simulink model "lars"  (R2021a)
settings: Solver=ode23s  StartTime=0.0  StopTime=10  FixedStep=0.5  RelTol=1e-3
values from neighbouring files (symbols this model uses):
  model =     [untitled.mat]
settings Model: Creator=niezhiwei  LastModifiedBy=niezhiwei
settings SolverCC: ConsecutiveZCsStepRelTol=eps
settings DataIOCC: SaveFinalState=on  SaveFormat=Array  ReturnWorkspaceOutputs=off  SignalLoggingName=sigsout

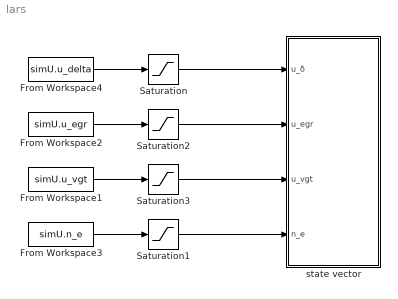
== system lars ==
  From Workspace1 : FromWorkspace  VariableName=simU.u_vgt  Interpolate=off  OutputAfterFinalValue=Holding final value
  From Workspace2 : FromWorkspace  VariableName=simU.u_egr  Interpolate=off  OutputAfterFinalValue=Holding final value
  From Workspace3 : FromWorkspace  VariableName=simU.n_e  Interpolate=off  OutputAfterFinalValue=Holding final value
  From Workspace4 : FromWorkspace  VariableName=simU.u_delta  Interpolate=off  OutputAfterFinalValue=Holding final value
  Saturation : Saturate  UpperLimit=250  LowerLimit=1
  Saturation1 : Saturate  UpperLimit=2000  LowerLimit=500
  Saturation2 : Saturate  UpperLimit=100  LowerLimit=0
  Saturation3 : Saturate  UpperLimit=100  LowerLimit=20
  state vector : Subsystem
  wires:
  Saturation/1 -> state vector/1(u_δ)
  From Workspace4/1 -> Saturation/1
  From Workspace3/1 -> Saturation1/1
  Saturation1/1 -> state vector/4(n_e)
  Saturation2/1 -> state vector/2(u_egr)
  From Workspace2/1 -> Saturation2/1
  Saturation3/1 -> state vector/3(u_vgt)
  From Workspace1/1 -> Saturation3/1

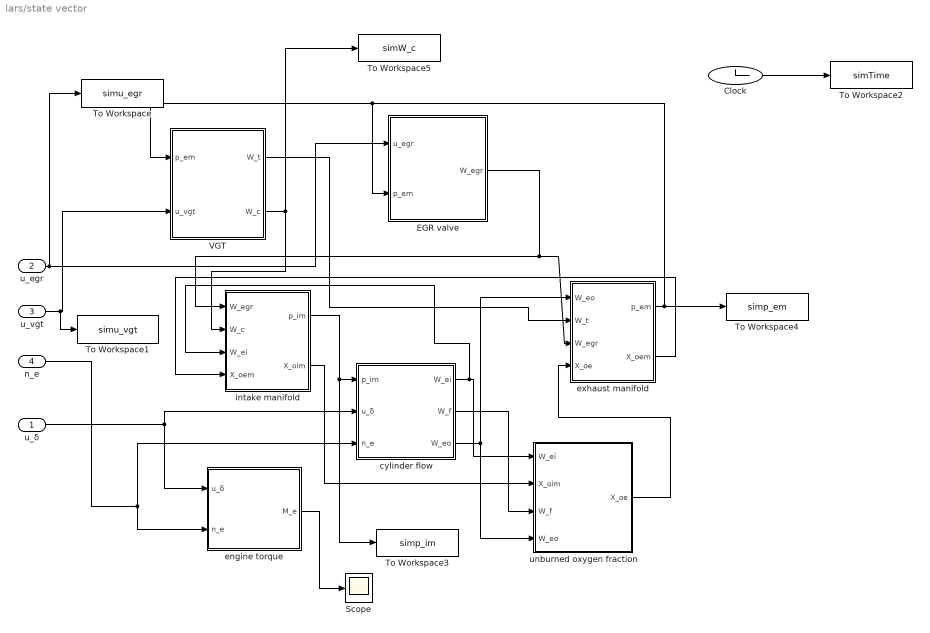
== system lars/state vector ==
  u_δ : Inport
  u_egr : Inport  Port=2
  u_vgt : Inport  Port=3
  n_e : Inport  Port=4
  Clock : Clock
  EGR valve : Subsystem
  Scope : Scope
  To Workspace : ToWorkspace  VariableName=simu_egr  SampleTime=-1
  To Workspace1 : ToWorkspace  VariableName=simu_vgt  SampleTime=-1
  To Workspace2 : ToWorkspace  VariableName=simTime  SampleTime=-1
  To Workspace3 : ToWorkspace  VariableName=simp_im  SampleTime=-1
  To Workspace4 : ToWorkspace  VariableName=simp_em  SampleTime=-1
  To Workspace5 : ToWorkspace  VariableName=simW_c  SampleTime=-1
  VGT : Subsystem
  cylinder flow : Subsystem
  engine torque : Subsystem
  exhaust manifold : Subsystem
  intake manifold : Subsystem
  unburned oxygen fraction : Subsystem
  wires:
  exhaust manifold/2(X_oem) -> intake manifold/4(X_oem)
  u_δ/1 -> engine torque/1(u_δ), cylinder flow/2(u_δ)
  n_e/1 -> engine torque/2(n_e), cylinder flow/3(n_e)
  cylinder flow/2(W_f) -> unburned oxygen fraction/3(W_f)
  intake manifold/2(X_oim) -> unburned oxygen fraction/2(X_oim)
  cylinder flow/1(W_ei) -> unburned oxygen fraction/1(W_ei), intake manifold/3(W_ei)
  cylinder flow/3(W_eo) -> exhaust manifold/1(W_eo), unburned oxygen fraction/4(W_eo)
  EGR valve/1(W_egr) -> intake manifold/1(W_egr), exhaust manifold/3(W_egr)
  VGT/1(W_t) -> exhaust manifold/2(W_t)
  u_vgt/1 -> To Workspace1/1, VGT/2(u_vgt)
  VGT/2(W_c) -> To Workspace5/1, intake manifold/2(W_c)
  unburned oxygen fraction/1(X_oe) -> exhaust manifold/4(X_oe)
  u_egr/1 -> To Workspace/1, EGR valve/1(u_egr)
  Clock/1 -> To Workspace2/1
  intake manifold/1(p_im) -> To Workspace3/1, cylinder flow/1(p_im)
  exhaust manifold/1(p_em) -> EGR valve/2(p_em), VGT/1(p_em), To Workspace4/1
  engine torque/1(M_e) -> Scope/1

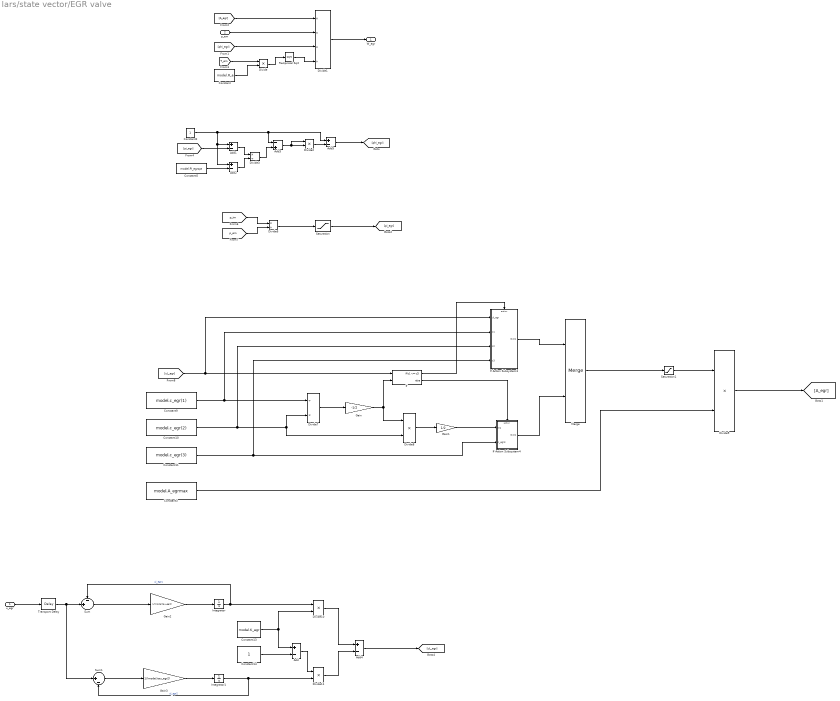
== system lars/state vector/EGR valve ==
  u_egr : Inport
  p_em : Inport  Port=2
  Add{,1..2,4..5} (5 alike) : Sum  Inputs=+-
  Add3 : Sum  Inputs=-+
  Constant : Constant  Value=model.R_e
  Constant10 : Constant  Value=model.c_egr(2)
  Constant11 : Constant  Value=model.c_egr(3)
  Constant13 : Constant  Value=model.K_egr
  Constant14 : Constant
  Constant2 : Constant
  Constant3 : Constant  Value=model.A_egrmax
  Constant5 : Constant  Value=model.PI_egropt
  Constant9 : Constant  Value=model.c_egr(1)
  Divide{,2,8..11} (6 alike) : Product  Inputs=**
  Divide1 : Product  Inputs=***/
  Divide3 : Product  Inputs=*/
  Divide6 : Product  Inputs=*/
  Divide7 : Product  Inputs=/*
  Gain : Gain  Gain=-1/2
  Gain1 : Gain  Gain=1/2
  Gain2 : Gain  Gain=1/(model.tau_egr1)
  Gain3 : Gain  Gain=1/(model.tau_egr2)
  If : If  NumInputs=2  IfExpression=u1 <= u2
  If Action Subsystem3 : Subsystem  TreatAsAtomicUnit=on
  If Action Subsystem4 : Subsystem  TreatAsAtomicUnit=on
  Integrator : Integrator  InitialCondition=model.uInit_egr
  Integrator1 : Integrator  InitialCondition=model.uInit_egr
  Merge : Merge
  Reciprocal Sqrt : Sqrt  SaturateOnIntegerOverflow=on
  Saturation : Saturate  UpperLimit=1  LowerLimit=model.PI_egropt
  Saturation1 : Saturate  UpperLimit=inf  LowerLimit=0
  Sum : Sum  Inputs=-+|
  Sum1 : Sum  Inputs=|+-
  Transport Delay : TransportDelay  DelayTime=model.tau_degr  InitialOutput=model.uInit_egr
  W_egr : Outport
  wires:
  [T_em] -> Divide/1
  Constant/1 -> Divide/2
  Divide/1 -> Reciprocal Sqrt/1
  [phi_egr] -> Divide1/3
  p_em/1 -> Divide1/2
  [A_egr] -> Divide1/1
  Reciprocal Sqrt/1 -> Divide1/4
  [pi_egr] -> Add1/2
  Constant2/1 -> Add2/1, Add1/1, Add5/1, Add3/1
  Constant5/1 -> Add2/2
  Add2/1 -> Divide3/2
  Add1/1 -> Divide3/1
  Divide3/1 -> Add3/2
  Add3/1 -> Divide2/1, Divide2/2
  Divide2/1 -> Add5/2
  Add5/1 -> [phi_egr]
  [p_im] -> Divide6/1
  [p_em] -> Divide6/2
  Divide1/1 -> W_egr/1
  Constant10/1 -> If Action Subsystem3/3(c2), Divide7/2, Divide8/2
  Constant9/1 -> If Action Subsystem3/2(c1), Divide7/1
  Divide7/1 -> Gain/1
  Gain/1 -> If/2, Divide8/1
  [uL_egr] -> If Action Subsystem3/1(ul_egr), If/1
  Constant11/1 -> If Action Subsystem3/4(c3), If Action Subsystem4/2(c_egr3)
  Divide8/1 -> Gain1/1
  Gain1/1 -> If Action Subsystem4/1(In1)
  Constant3/1 -> Divide9/2
  Divide9/1 -> [A_egr]
  Integrator/1 -> Divide10/1, Sum/1  "ul_egr1"
  Constant13/1 -> Add/1, Divide10/2
  Constant14/1 -> Add/2
  Integrator1/1 -> Sum1/2, Divide11/2  "ul_egr2"
  Add/1 -> Divide11/1
  Divide10/1 -> Add4/1
  Divide11/1 -> Add4/2
  Add4/1 -> [uL_egr]
  Gain2/1 -> Integrator/1
  Sum/1 -> Gain2/1
  Sum1/1 -> Gain3/1
  Gain3/1 -> Integrator1/1
  u_egr/1 -> Transport Delay/1
  Transport Delay/1 -> Sum/2, Sum1/1
  Saturation/1 -> [pi_egr]
  Divide6/1 -> Saturation/1
  If/2 -> If Action Subsystem4/Action
  If/1 -> If Action Subsystem3/Action
  Merge/1 -> Saturation1/1
  If Action Subsystem3/1(Out1) -> Merge/1
  If Action Subsystem4/1(Out1) -> Merge/2
  Saturation1/1 -> Divide9/1

== system lars/state vector/VGT ==
  p_em : Inport
  u_vgt : Inport  Port=2
  To Workspace3 : ToWorkspace  VariableName=W_c  SampleTime=-1
  compressor : Subsystem
  turbo : Subsystem
  W_t : Outport
  W_c : Outport  Port=2
  wires:
  turbo/1(W_t) -> W_t/1
  u_vgt/1 -> turbo/1(u_vgt)
  compressor/1(W_c) -> W_c/1, To Workspace3/1
  turbo/2(omega_t) -> compressor/1(omega_t)
  p_em/1 -> turbo/2(p_em)
  compressor/2(P_c) -> turbo/3(P_c)

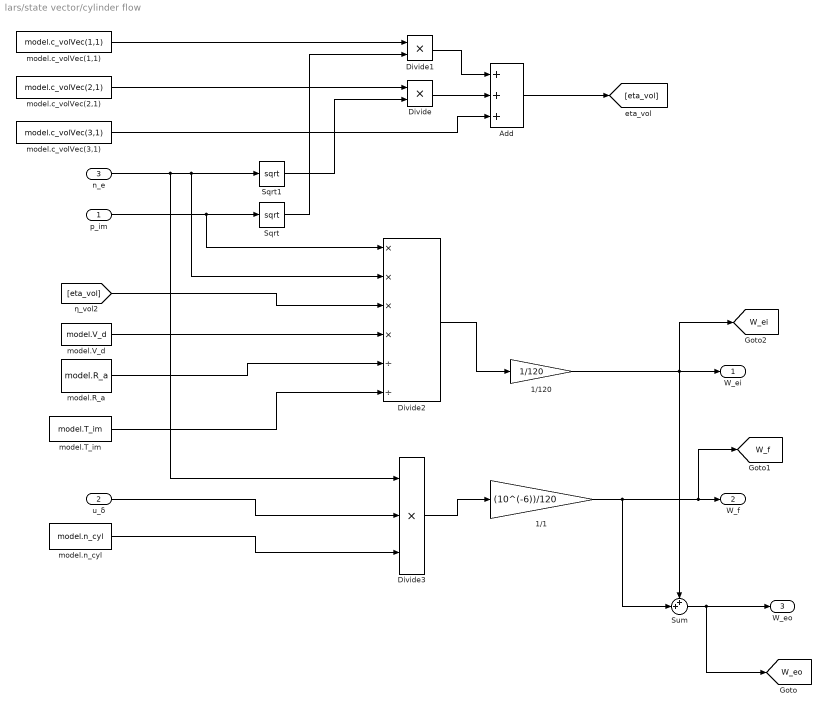
== system lars/state vector/cylinder flow ==
  p_im : Inport
  u_δ : Inport  Port=2
  n_e : Inport  Port=3
  1/1 : Gain  Gain=(10^(-6))/120
  1/120 : Gain  Gain=1/120
  Add : Sum  Inputs=+++
  Divide : Product  Inputs=**
  Divide1 : Product  Inputs=**
  Divide2 : Product  Inputs=****//
  Divide3 : Product  Inputs=***
  Sqrt : Sqrt  SaturateOnIntegerOverflow=on
  Sqrt1 : Sqrt  SaturateOnIntegerOverflow=on
  Sum : Sum  Inputs=++|
  model.R_a : Constant  Value=model.R_a
  model.T_im : Constant  Value=model.T_im
  model.V_d : Constant  Value=model.V_d
  model.c_volVec(1,1) : Constant  Value=model.c_volVec(1,1)
  model.c_volVec(2,1) : Constant  Value=model.c_volVec(2,1)
  model.c_volVec(3,1) : Constant  Value=model.c_volVec(3,1)
  model.n_cyl : Constant  Value=model.n_cyl
  W_ei : Outport
  W_f : Outport  Port=2
  W_eo : Outport  Port=3
  tag scope: W_ei=global, W_eo=global, W_f=global
  wires:
  p_im/1 -> Divide2/1, Sqrt/1
  n_e/1 -> Divide3/1, Divide2/2, Sqrt1/1
  model.c_volVec(2,1)/1 -> Divide/1
  model.c_volVec(1,1)/1 -> Divide1/1
  Sqrt/1 -> Divide1/2
  Divide1/1 -> Add/1
  Divide/1 -> Add/2
  model.c_volVec(3,1)/1 -> Add/3
  Add/1 -> [eta_vol]
  [eta_vol] -> Divide2/3
  model.V_d/1 -> Divide2/4
  model.R_a/1 -> Divide2/5
  model.T_im/1 -> Divide2/6
  Divide2/1 -> 1/120/1
  1/120/1 -> [W_ei], Sum/1, W_ei/1
  u_δ/1 -> Divide3/2
  model.n_cyl/1 -> Divide3/3
  Divide3/1 -> 1/1/1
  1/1/1 -> Sum/2, [W_f], W_f/1
  Sum/1 -> [W_eo], W_eo/1
  Sqrt1/1 -> Divide/2

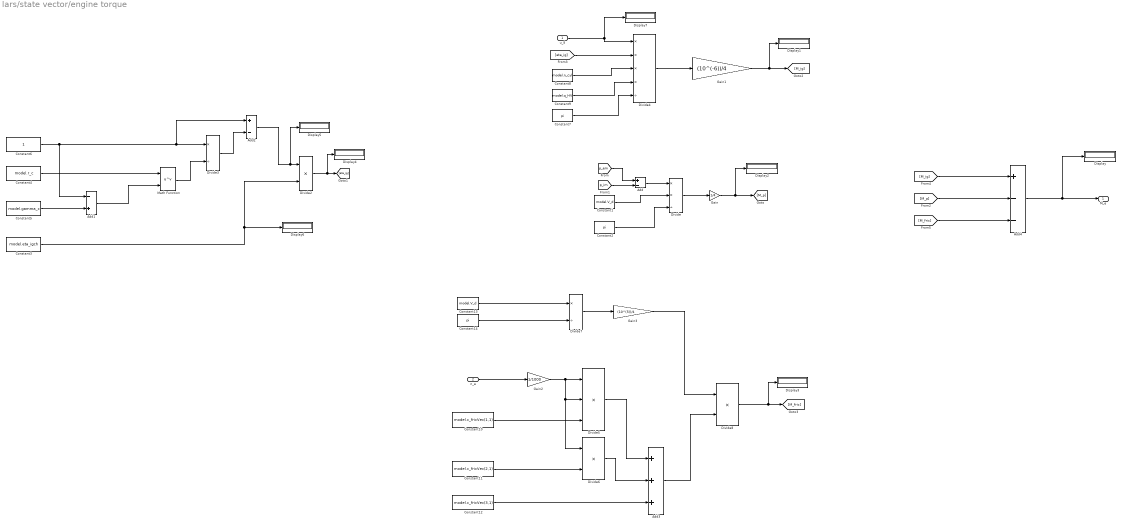
== system lars/state vector/engine torque ==
  u_δ : Inport
  n_e : Inport  Port=2
  Add : Sum  Inputs=+-
  Add1 : Sum  Inputs=-+
  Add2 : Sum  Inputs=+-
  Add3 : Sum  Inputs=+++
  Add4 : Sum  Inputs=+--
  Constant1 : Constant  Value=model.V_d
  Constant10 : Constant  Value=model.c_fricVec(1,1)
  Constant11 : Constant  Value=model.c_fricVec(2,1)
  Constant12 : Constant  Value=model.c_fricVec(3,1)
  Constant13 : Constant  Value=model.V_d
  Constant14 : Constant  Value=pi
  Constant2 : Constant  Value=pi
  Constant3 : Constant  Value=model.eta_igch
  Constant4 : Constant  Value=model.r_c
  Constant5 : Constant  Value=model.gamma_c
  Constant6 : Constant
  Constant7 : Constant  Value=pi
  Constant8 : Constant  Value=model.n_cyl
  Constant9 : Constant  Value=model.q_HV
  Display{,1..7} (8 alike) : Display
  Divide : Product  Inputs=**/
  Divide2 : Product  Inputs=**
  Divide3 : Product  Inputs=*/
  Divide4 : Product  Inputs=****/
  Divide5 : Product  Inputs=***
  Divide6 : Product  Inputs=**
  Divide7 : Product  Inputs=*/
  Divide8 : Product  Inputs=**
  Gain : Gain  Gain=1/4
  Gain1 : Gain  Gain=(10^(-6))/4
  Gain2 : Gain  Gain=1/1000
  Gain3 : Gain  Gain=(10^(5))/4
  Math Function : Math  Operator=pow  SaturateOnIntegerOverflow=on
  M_e : Outport
  wires:
  [p_em] -> Add/1
  [p_im] -> Add/2
  Add/1 -> Divide/1
  Constant1/1 -> Divide/2
  Constant2/1 -> Divide/3
  Divide/1 -> Gain/1
  Constant6/1 -> Add1/1, Add2/1, Divide3/1
  Constant4/1 -> Math Function/1
  Math Function/1 -> Divide3/2
  Divide3/1 -> Add2/2
  Constant3/1 -> Display6/1, Divide2/2
  Add2/1 -> Display5/1, Divide2/1
  Divide2/1 -> Display4/1, [eta_ig]
  u_δ/1 -> Display7/1, Divide4/1
  [eta_ig] -> Divide4/2
  Constant8/1 -> Divide4/3
  Constant9/1 -> Divide4/4
  Constant7/1 -> Divide4/5
  Divide4/1 -> Gain1/1
  Gain1/1 -> Display1/1, [M_ig]
  n_e/1 -> Gain2/1
  Gain2/1 -> Divide5/1, Divide5/2, Divide6/1
  Constant10/1 -> Divide5/3
  Constant11/1 -> Divide6/2
  Divide5/1 -> Add3/1
  Divide6/1 -> Add3/2
  Constant12/1 -> Add3/3
  Constant13/1 -> Divide7/1
  Constant14/1 -> Divide7/2
  Divide7/1 -> Gain3/1
  Gain3/1 -> Divide8/1
  Add3/1 -> Divide8/2
  Divide8/1 -> Display3/1, [M_fric]
  [M_ig] -> Add4/1
  [M_p] -> Add4/2
  [M_fric] -> Add4/3
  Add4/1 -> Display/1, M_e/1
  Gain/1 -> Display2/1, [M_p]
  Constant5/1 -> Add1/2
  Add1/1 -> Math Function/2

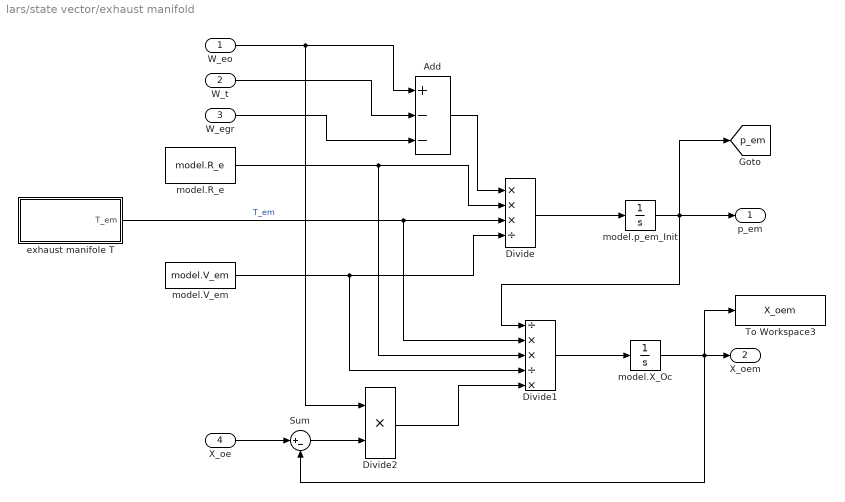
== system lars/state vector/exhaust manifold ==
  W_eo : Inport
  W_t : Inport  Port=2
  W_egr : Inport  Port=3
  X_oe : Inport  Port=4
  Add : Sum  Inputs=+--
  Divide : Product  Inputs=***/
  Divide1 : Product  Inputs=/**/*
  Divide2 : Product  Inputs=**
  Sum : Sum  Inputs=|+-
  To Workspace3 : ToWorkspace  VariableName=X_oem  SampleTime=-1
  exhaust manifole T : Subsystem
  model.R_e : Constant  Value=model.R_e
  model.V_em : Constant  Value=model.V_em
  model.X_Oc : Integrator  LimitOutput=on  UpperSaturationLimit=1  LowerSaturationLimit=0
  model.p_em_Init : Integrator  InitialCondition=model.p_em_Init  LimitOutput=on  UpperSaturationLimit=20*model.p_amb  LowerSaturationLimit=0.5*model.p_amb
  p_em : Outport
  X_oem : Outport  Port=2
  tag scope: p_em=global
  wires:
  model.p_em_Init/1 -> Divide1/1, [p_em], p_em/1
  model.R_e/1 -> Divide1/3, Divide/2
  exhaust manifole T/1(T_em) -> Divide/3, Divide1/2  "T_em"
  model.V_em/1 -> Divide1/4, Divide/4
  Add/1 -> Divide/1
  W_egr/1 -> Add/3
  W_t/1 -> Add/2
  W_eo/1 -> Add/1, Divide2/1
  Divide1/1 -> model.X_Oc/1
  X_oe/1 -> Sum/1
  Divide2/1 -> Divide1/5
  Sum/1 -> Divide2/2
  Divide/1 -> model.p_em_Init/1
  model.X_Oc/1 -> To Workspace3/1, Sum/2, X_oem/1

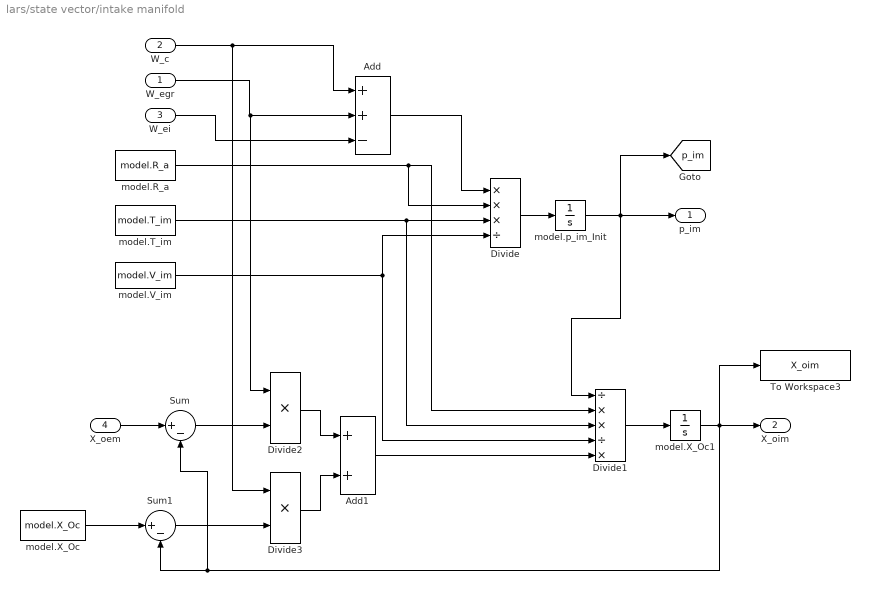
== system lars/state vector/intake manifold ==
  W_egr : Inport
  W_c : Inport  Port=2
  W_ei : Inport  Port=3
  X_oem : Inport  Port=4
  Add : Sum  Inputs=++-
  Add1 : Sum
  Divide : Product  Inputs=***/
  Divide1 : Product  Inputs=/**/*
  Divide2 : Product  Inputs=**
  Divide3 : Product  Inputs=**
  Sum : Sum  Inputs=|+-
  Sum1 : Sum  Inputs=|+-
  To Workspace3 : ToWorkspace  VariableName=X_oim  SampleTime=-1
  model.R_a : Constant  Value=model.R_a
  model.T_im : Constant  Value=model.T_im
  model.V_im : Constant  Value=model.V_im
  model.X_Oc : Constant  Value=model.X_Oc
  model.X_Oc1 : Integrator  LimitOutput=on  UpperSaturationLimit=1  LowerSaturationLimit=0
  model.p_im_Init : Integrator  InitialCondition=model.p_im_Init  LimitOutput=on  UpperSaturationLimit=10*model.p_amb  LowerSaturationLimit=0.5*model.p_amb
  p_im : Outport
  X_oim : Outport  Port=2
  tag scope: p_im=global
  wires:
  W_egr/1 -> Divide2/1, Add/2
  W_ei/1 -> Add/3
  Add/1 -> Divide/1
  model.V_im/1 -> Divide/4, Divide1/4
  model.T_im/1 -> Divide/3, Divide1/3
  model.R_a/1 -> Divide1/2, Divide/2
  Divide/1 -> model.p_im_Init/1
  model.p_im_Init/1 -> Divide1/1, [p_im], p_im/1
  Divide1/1 -> model.X_Oc1/1
  X_oem/1 -> Sum/1
  model.X_Oc/1 -> Sum1/1
  Sum/1 -> Divide2/2
  Sum1/1 -> Divide3/2
  Divide2/1 -> Add1/1
  Divide3/1 -> Add1/2
  Add1/1 -> Divide1/5
  W_c/1 -> Add/1, Divide3/1
  model.X_Oc1/1 -> To Workspace3/1, Sum1/2, Sum/2, X_oim/1

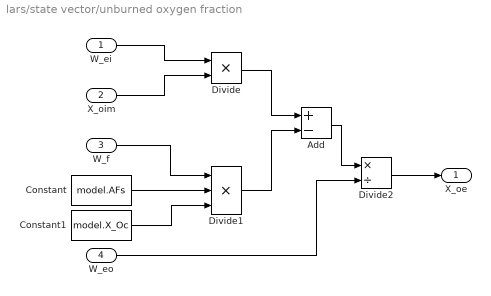
== system lars/state vector/unburned oxygen fraction ==
  W_ei : Inport
  X_oim : Inport  Port=2
  W_f : Inport  Port=3
  W_eo : Inport  Port=4
  Add : Sum  Inputs=+-
  Constant : Constant  Value=model.AFs
  Constant1 : Constant  Value=model.X_Oc
  Divide : Product  Inputs=**
  Divide1 : Product  Inputs=***
  Divide2 : Product  Inputs=*/
  X_oe : Outport
  wires:
  X_oim/1 -> Divide/2
  W_f/1 -> Divide1/1
  Constant/1 -> Divide1/2
  Divide/1 -> Add/1
  Divide1/1 -> Add/2
  Add/1 -> Divide2/1
  W_eo/1 -> Divide2/2
  Divide2/1 -> X_oe/1
  W_ei/1 -> Divide/1
  Constant1/1 -> Divide1/3

== system lars/state vector/EGR valve/If Action Subsystem3 ==
  ul_egr : Inport
  c1 : Inport  Port=2
  c2 : Inport  Port=3
  c3 : Inport  Port=4
  Action Port : ActionPort  ActionPortLabel=if(u1 <= u2)
  Add : Sum  Inputs=+++
  Divide : Product  Inputs=***
  Divide1 : Product  Inputs=**
  Out1 : Outport
  wires:
  ul_egr/1 -> Divide1/1, Divide/2, Divide/1
  c1/1 -> Divide/3
  c2/1 -> Divide1/2
  Divide/1 -> Add/1
  Divide1/1 -> Add/2
  c3/1 -> Add/3
  Add/1 -> Out1/1

== system lars/state vector/EGR valve/If Action Subsystem4 ==
  In1 : Inport
  c_egr3 : Inport  Port=2
  Action Port : ActionPort  ActionPortLabel=else
  Add : Sum
  Out1 : Outport
  wires:
  In1/1 -> Add/1
  c_egr3/1 -> Add/2
  Add/1 -> Out1/1

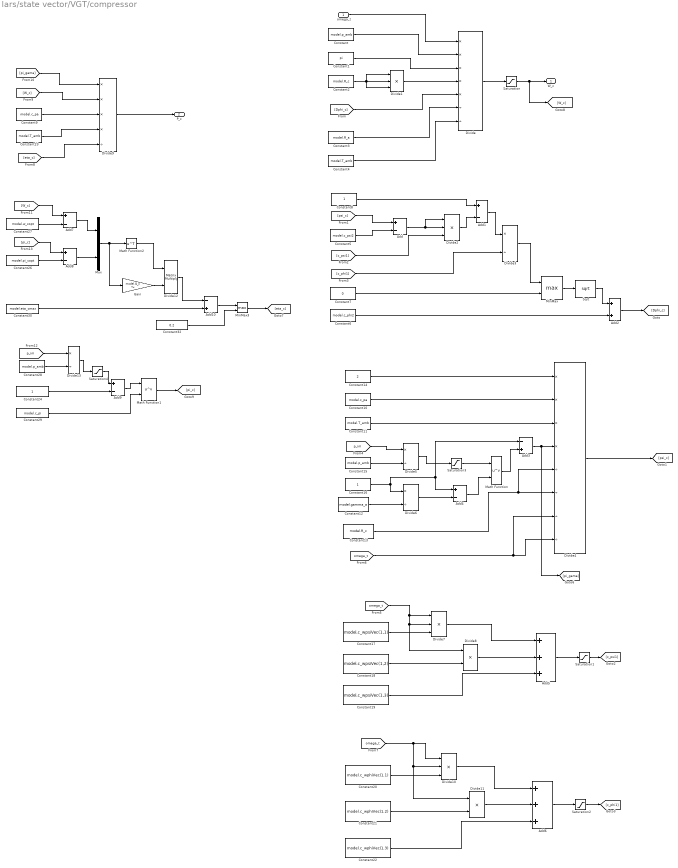
== system lars/state vector/VGT/compressor ==
  omega_t : Inport
  Add{,1,4,7..9} (6 alike) : Sum  Inputs=+-
  Add10 : Sum  Inputs=-+
  Add2 : Sum
  Add3 : Sum  Inputs=-+
  Add5 : Sum  Inputs=+++
  Add6 : Sum  Inputs=+++
  Constant : Constant  Value=model.p_amb
  Constant1 : Constant  Value=pi
  Constant10 : Constant  Value=model.c_pa
  Constant11 : Constant  Value=model.T_amb
  Constant12 : Constant  Value=model.gamma_a
  Constant13 : Constant  Value=model.R_c
  Constant14 : Constant  Value=2
  Constant15 : Constant  Value=model.p_amb
  Constant16 : Constant
  Constant17 : Constant  Value=model.c_wpsiVec(1,1)
  Constant18 : Constant  Value=model.c_wpsiVec(1,2)
  Constant19 : Constant  Value=model.c_wpsiVec(1,3)
  Constant2 : Constant  Value=model.R_c
  Constant20 : Constant  Value=model.c_wphiVec(1,1)
  Constant21 : Constant  Value=model.c_wphiVec(1,2)
  Constant22 : Constant  Value=model.c_wphiVec(1,3)
  Constant23 : Constant  Value=model.T_amb
  Constant24 : Constant
  Constant26 : Constant  Value=model.pi_copt
  Constant27 : Constant  Value=model.w_copt
  Constant28 : Constant  Value=model.p_amb
  Constant29 : Constant  Value=model.c_pi
  Constant3 : Constant  Value=model.R_a
  Constant30 : Constant  Value=model.eta_cmax
  Constant32 : Constant  Value=0.2
  Constant4 : Constant  Value=model.T_amb
  Constant5 : Constant  Value=model.c_psi2
  Constant6 : Constant  Value=model.c_phi2
  Constant7 : Constant  Value=0
  Constant8 : Constant
  Constant9 : Constant  Value=model.c_pa
  Divide : Product  Inputs=*****//
  Divide{1..2,7,10} (4 alike) : Product  Inputs=***
  Divide11 : Product  Inputs=**
  Divide12 : Product  Inputs=**  Multiplication=Matrix(*)
  Divide{3,5..6,13} (4 alike) : Product  Inputs=*/
  Divide4 : Product  Inputs=****////
  Divide8 : Product  Inputs=**
  Divide9 : Product  Inputs=****/
  Gain : Gain  Gain=model.Q_c  Multiplication=Matrix(K*u)
  Math Function : Math  Operator=pow  SaturateOnIntegerOverflow=on
  Math Function1 : Math  Operator=pow  SaturateOnIntegerOverflow=on
  Math Function2 : Math  Operator=transpose  SaturateOnIntegerOverflow=on
  MinMax : MinMax  Function=max  Inputs=2
  MinMax3 : MinMax  Function=max  Inputs=2
  Mux : Mux  Inputs=2
  Saturation : Saturate  UpperLimit=inf  LowerLimit=1e-4
  Saturation1 : Saturate  UpperLimit=inf  LowerLimit=0
  Saturation2 : Saturate  UpperLimit=inf  LowerLimit=0.1
  Saturation3 : Saturate  UpperLimit=inf  LowerLimit=1
  Saturation4 : Saturate  UpperLimit=inf  LowerLimit=1
  Sqrt : Sqrt  SaturateOnIntegerOverflow=on
  W_c : Outport
  P_c : Outport  Port=2
  wires:
  Constant2/1 -> Divide1/3, Divide1/1, Divide1/2
  Divide1/1 -> Divide/4
  Constant1/1 -> Divide/3
  Constant/1 -> Divide/2
  omega_t/1 -> Divide/1
  [Dphi_c] -> Divide/5
  Constant3/1 -> Divide/6
  MinMax/1 -> Sqrt/1
  Constant5/1 -> Add/2
  [psi_c] -> Add/1
  Add/1 -> Divide2/1, Divide2/2
  [c_psi1] -> Divide2/3
  Constant8/1 -> Add1/1
  Divide2/1 -> Add1/2
  Add1/1 -> Divide3/1
  [c_phi1] -> Divide3/2
  Divide3/1 -> MinMax/1
  Constant7/1 -> MinMax/2
  Sqrt/1 -> Add2/1
  Constant6/1 -> Add2/2
  Add2/1 -> [Dphi_c]
  [p_im] -> Divide5/1
  Constant15/1 -> Divide5/2
  Constant16/1 -> Add3/1, Add4/1, Divide6/1
  Constant12/1 -> Divide6/2
  Divide6/1 -> Add4/2
  Add4/1 -> Math Function/2
  Math Function/1 -> Add3/2
  Add3/1 -> Divide4/4, [pi_gama]
  Constant11/1 -> Divide4/3
  Constant10/1 -> Divide4/2
  Constant14/1 -> Divide4/1
  Constant13/1 -> Divide4/5, Divide4/6
  [omega_t] -> Divide4/7, Divide4/8
  Divide4/1 -> [psi_c]
  Constant17/1 -> Divide7/3
  [omega_t] -> Divide7/1, Divide8/1, Divide7/2
  Constant18/1 -> Divide8/2
  Divide8/1 -> Add5/2
  Divide7/1 -> Add5/1
  Constant20/1 -> Divide10/3
  [omega_t] -> Divide11/1, Divide10/2, Divide10/1
  Constant21/1 -> Divide11/2
  Constant19/1 -> Add5/3
  Divide11/1 -> Add6/2
  Constant22/1 -> Add6/3
  Divide10/1 -> Add6/1
  [eta_c] -> Divide9/5
  Constant23/1 -> Divide9/4
  Constant9/1 -> Divide9/3
  [W_c] -> Divide9/2
  [pi_gama] -> Divide9/1
  Divide9/1 -> P_c/1
  Constant27/1 -> Add7/2
  [W_c] -> Add7/1
  Constant26/1 -> Add8/2
  [pi_c] -> Add8/1
  Add8/1 -> Mux/2
  Add7/1 -> Mux/1
  [p_im] -> Divide13/1
  Constant28/1 -> Divide13/2
  Constant24/1 -> Add9/2
  Add9/1 -> Math Function1/1
  Constant29/1 -> Math Function1/2
  Math Function1/1 -> [pi_c]
  Divide12/1 -> Add10/1
  Constant30/1 -> Add10/2
  Add10/1 -> MinMax3/1
  Divide13/1 -> Saturation4/1
  Constant32/1 -> MinMax3/2
  MinMax3/1 -> [eta_c]
  Divide/1 -> Saturation/1
  Saturation/1 -> [W_c], W_c/1
  Saturation1/1 -> [c_psi1]
  Add5/1 -> Saturation1/1
  Saturation2/1 -> [c_phi1]
  Add6/1 -> Saturation2/1
  Saturation3/1 -> Math Function/1
  Divide5/1 -> Saturation3/1
  Saturation4/1 -> Add9/1
  Mux/1 -> Gain/1, Math Function2/1
  Gain/1 -> Divide12/2
  Math Function2/1 -> Divide12/1
  Constant4/1 -> Divide/7

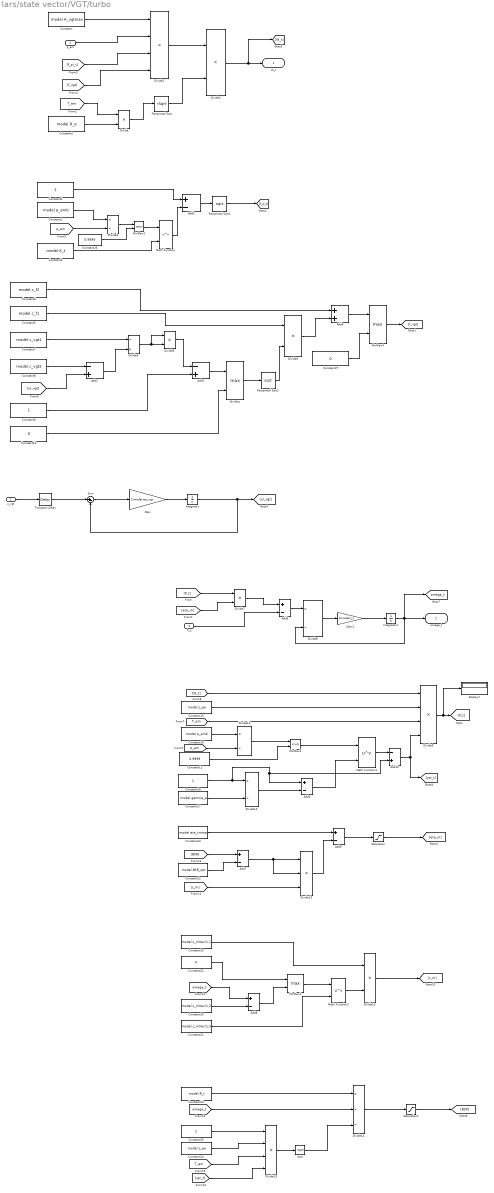
== system lars/state vector/VGT/turbo ==
  u_vgt : Inport
  p_em : Inport  Port=2
  P_c : Inport  Port=3
  Add{1,5..9} (6 alike) : Sum  Inputs=+-
  Add10 : Sum  Inputs=-+
  Add2 : Sum  Inputs=-+
  Add3 : Sum  Inputs=-+
  Add4 : Sum
  Constant : Constant  Value=model.A_vgtmax
  Constant1 : Constant  Value=model.p_amb
  Constant10 : Constant  Value=0
  Constant11 : Constant  Value=0.9999
  Constant12 : Constant  Value=model.BSR_opt
  Constant13 : Constant  Value=model.eta_tmmax
  Constant15 : Constant  Value=model.c_pe
  Constant16 : Constant  Value=model.p_amb
  Constant17 : Constant  Value=model.gamma_e
  Constant18 : Constant
  Constant19 : Constant  Value=model.c_mVec(1,1)
  Constant2 : Constant  Value=model.R_e
  Constant20 : Constant  Value=model.c_mVec(1,2)
  Constant21 : Constant  Value=model.c_mVec(1,3)
  Constant22 : Constant  Value=0
  Constant23 : Constant  Value=model.R_t
  Constant24 : Constant  Value=model.c_pe
  Constant25 : Constant  Value=2
  Constant26 : Constant  Value=0.9999
  Constant27 : Constant  Value=0
  Constant3 : Constant  Value=model.K_t
  Constant4 : Constant
  Constant5 : Constant  Value=model.c_f1
  Constant6 : Constant  Value=model.c_f2
  Constant7 : Constant  Value=model.c_vgt1
  Constant8 : Constant  Value=model.c_vgt2
  Constant9 : Constant
  Display7 : Display
  Divide{,2,5..7,10} (6 alike) : Product  Inputs=**
  Divide1 : Product  Inputs=****
  Divide{3,8,11..12} (4 alike) : Product  Inputs=*/
  Divide13 : Product  Inputs=***
  Divide14 : Product  Inputs=**/
  Divide15 : Product  Inputs=****
  Divide4 : Product  Inputs=/*
  Divide9 : Product  Inputs=****
  Gain : Gain  Gain=1/model.tau_vgt
  Gain1 : Gain  Gain=1/model.J_t
  Integrator : Integrator  InitialCondition=model.uInit_vgt
  Integrator1 : Integrator  InitialCondition=model.omega_t_Init  LimitOutput=on  UpperSaturationLimit=200000*pi/30  LowerSaturationLimit=100*pi/30
  Math Function : Math  Operator=pow  SaturateOnIntegerOverflow=on
  Math Function1 : Math  Operator=pow  SaturateOnIntegerOverflow=on
  Math Function2 : Math  Operator=pow  SaturateOnIntegerOverflow=on
  MinMax : MinMax  Function=max  Inputs=2
  MinMax1 : MinMax  Function=max  Inputs=2
  MinMax2 : MinMax  Inputs=2
  MinMax3 : MinMax  Inputs=2
  MinMax4 : MinMax  Function=max  Inputs=2
  Reciprocal Sqrt : Sqrt  Operator=rSqrt  SaturateOnIntegerOverflow=on
  Reciprocal Sqrt1 : Sqrt  SaturateOnIntegerOverflow=on
  Reciprocal Sqrt2 : Sqrt  SaturateOnIntegerOverflow=on
  Saturation : Saturate  UpperLimit=1  LowerLimit=0.2
  Saturation1 : Saturate  UpperLimit=2*model.BSR_opt  LowerLimit=0
  Sqrt : Sqrt  SaturateOnIntegerOverflow=on
  Sum : Sum  Inputs=|+-
  Transport Delay : TransportDelay  DelayTime=model.tau_dvgt  InitialOutput=model.uInit_vgt
  W_t : Outport
  omega_t : Outport  Port=2
  tag scope: omega_t=global
  wires:
  Integrator/1 -> Sum/2, [ul_vgt]
  Add1/1 -> Reciprocal Sqrt1/1
  MinMax/1 -> Reciprocal Sqrt2/1
  Transport Delay/1 -> Sum/1
  Divide4/1 -> Divide5/1, Divide5/2
  Constant10/1 -> MinMax/2
  [T_em] -> Divide/1
  Divide6/1 -> Add4/2
  Divide/1 -> Reciprocal Sqrt/1
  Constant2/1 -> Divide/2
  [ul_vgt] -> Add2/2
  Add3/1 -> MinMax/1
  Sum/1 -> Gain/1
  Constant4/1 -> Add1/1
  Math Function/1 -> Add1/2
  Reciprocal Sqrt1/1 -> [f_pi_t]
  [p_em] -> Divide3/2
  Constant/1 -> Divide1/1
  Reciprocal Sqrt2/1 -> Divide6/2
  [f_pi_t] -> Divide1/3
  Divide5/1 -> Add3/1
  [f_vgt] -> Divide1/4
  Constant8/1 -> Add2/1
  p_em/1 -> Divide1/2
  Gain/1 -> Integrator/1
  Constant5/1 -> Divide6/1
  Reciprocal Sqrt/1 -> Divide2/2
  u_vgt/1 -> Transport Delay/1
  Constant9/1 -> Add3/2
  Constant3/1 -> Math Function/2
  Add2/1 -> Divide4/2
  Divide1/1 -> Divide2/1
  Constant6/1 -> Add4/1
  Constant7/1 -> Divide4/1
  Constant1/1 -> Divide3/1
  Divide2/1 -> [W_t], W_t/1
  Integrator1/1 -> Divide8/2, [omega_t], omega_t/1
  [P_t] -> Divide7/1
  [eta_m] -> Divide7/2
  P_c/1 -> Add5/2
  Divide7/1 -> Add5/1
  Add5/1 -> Divide8/1
  [W_t] -> Divide9/1
  Constant15/1 -> Divide9/2
  Constant16/1 -> Divide11/1
  Constant17/1 -> Divide12/2
  Divide12/1 -> Add6/2
  Add6/1 -> Math Function1/2
  [omega_t] -> Add8/1
  Constant20/1 -> Add8/2
  Add8/1 -> MinMax1/2
  Constant22/1 -> MinMax1/1
  MinMax1/1 -> Math Function2/1
  Constant21/1 -> Math Function2/2
  Math Function2/1 -> Divide10/2
  Constant19/1 -> Divide10/1
  Divide10/1 -> [c_m]
  [BSR] -> Add7/1
  Constant12/1 -> Add7/2
  [c_m] -> Divide13/3
  Add7/1 -> Divide13/2, Divide13/1
  Constant13/1 -> Add9/1
  Divide13/1 -> Add9/2
  Math Function1/1 -> Add10/1
  Add10/1 -> [ypi_t], Divide9/4
  Constant24/1 -> Divide15/2
  Constant25/1 -> Divide15/1
  [T_em] -> Divide15/3
  [ypi_t] -> Divide15/4
  Divide15/1 -> Sqrt/1
  Constant23/1 -> Divide14/1
  Sqrt/1 -> Divide14/3
  [T_em] -> Divide9/3
  Constant18/1 -> Add10/2, Add6/1, Divide12/1
  Divide9/1 -> Display7/1, [P_t]
  [omega_t] -> Divide14/2
  [p_em] -> Divide11/2
  Divide11/1 -> MinMax2/1
  MinMax2/1 -> Math Function1/1
  Constant11/1 -> MinMax2/2
  MinMax3/1 -> Math Function/1
  Divide3/1 -> MinMax3/1
  Constant26/1 -> MinMax3/2
  Add4/1 -> MinMax4/1
  Constant27/1 -> MinMax4/2
  MinMax4/1 -> [f_vgt]
  Saturation/1 -> [eta_m]
  Add9/1 -> Saturation/1
  Divide14/1 -> Saturation1/1
  Saturation1/1 -> [BSR]
  Gain1/1 -> Integrator1/1
  Divide8/1 -> Gain1/1

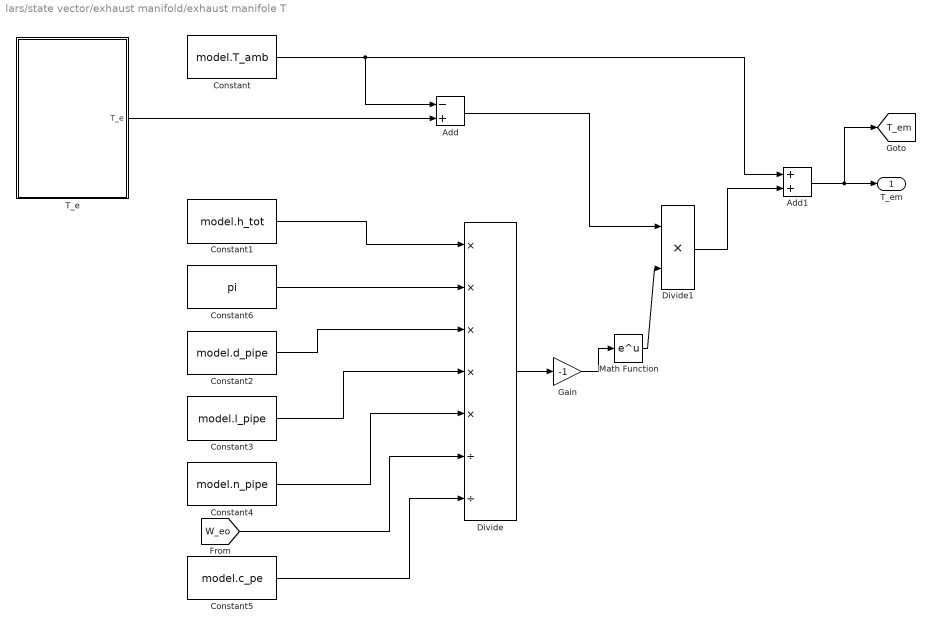
== system lars/state vector/exhaust manifold/exhaust manifole T ==
  Add : Sum  Inputs=-+
  Add1 : Sum
  Constant : Constant  Value=model.T_amb
  Constant1 : Constant  Value=model.h_tot
  Constant2 : Constant  Value=model.d_pipe
  Constant3 : Constant  Value=model.l_pipe
  Constant4 : Constant  Value=model.n_pipe
  Constant5 : Constant  Value=model.c_pe
  Constant6 : Constant  Value=pi
  Divide : Product  Inputs=*****//
  Divide1 : Product  Inputs=**
  Gain : Gain  Gain=-1
  Math Function : Math  SaturateOnIntegerOverflow=on
  T_e : Subsystem
  T_em : Outport
  tag scope: T_em=global
  wires:
  [W_eo] -> Divide/6
  Constant1/1 -> Divide/1
  Constant2/1 -> Divide/3
  Constant3/1 -> Divide/4
  Constant4/1 -> Divide/5
  Constant5/1 -> Divide/7
  Constant/1 -> Add1/1, Add/1
  Math Function/1 -> Divide1/2
  Add/1 -> Divide1/1
  Divide1/1 -> Add1/2
  Constant6/1 -> Divide/2
  T_e/1(T_e) -> Add/2
  Add1/1 -> [T_em], T_em/1
  Divide/1 -> Gain/1
  Gain/1 -> Math Function/1

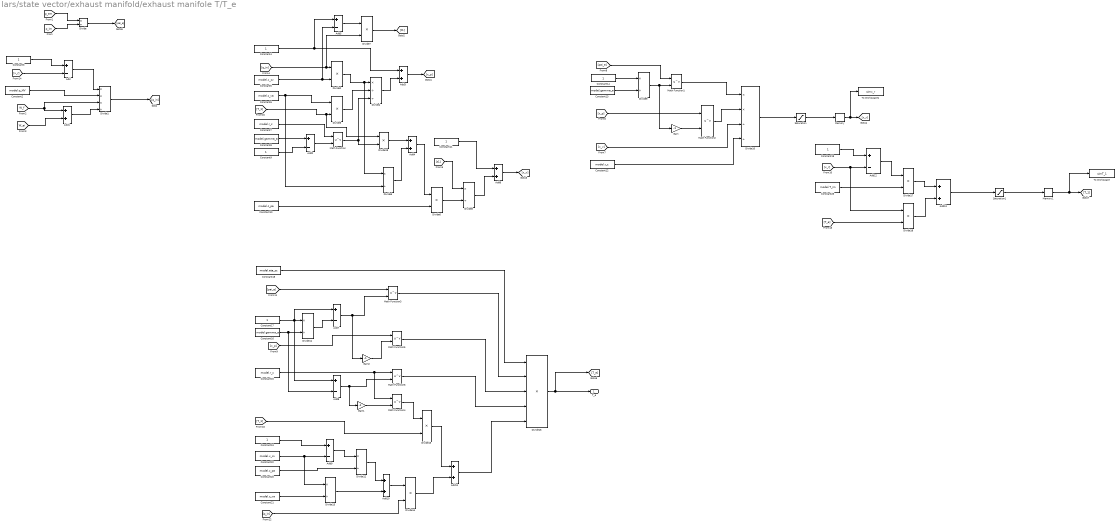
== system lars/state vector/exhaust manifold/exhaust manifole T/T_e ==
  Add{,2,5,7..9,12} (7 alike) : Sum  Inputs=+-
  Add{1,3..4,6,10..11,13} (7 alike) : Sum
  Constant10 : Constant  Value=model.c_pa
  Constant{3..4,9,11,14,17,19,24} (8 alike) : Constant
  Constant12 : Constant  Value=model.r_c
  Constant13 : Constant  Value=model.gamma_a
  Constant15 : Constant  Value=model.r_c
  Constant16 : Constant  Value=model.gamma_a
  Constant18 : Constant  Value=model.eta_sc
  Constant2 : Constant  Value=model.q_HV
  Constant20 : Constant  Value=model.c_pa
  Constant21 : Constant  Value=model.c_va
  Constant22 : Constant  Value=model.x_cv
  Constant25 : Constant  Value=model.T_im
  Constant5 : Constant  Value=model.x_cv
  Constant6 : Constant  Value=model.c_va
  Constant7 : Constant  Value=model.r_c
  Constant8 : Constant  Value=model.gamma_a
  Divide{,5,8..9,11..13} (7 alike) : Product  Inputs=*/
  Divide1 : Product  Inputs=***/
  Divide10 : Product  Inputs=**//
  Divide{2..3,6..7,14..15,17..19} (9 alike) : Product  Inputs=**
  Divide16 : Product  Inputs=*****
  Divide4 : Product  Inputs=*//
  Gain : Gain  Gain=-1
  Gain1 : Gain  Gain=-1
  Gain2 : Gain  Gain=-1
  Math Function{,1..6} (7 alike) : Math  Operator=pow  SaturateOnIntegerOverflow=on
  Memory : Memory  InitialCondition=model.x_r_Init  InheritSampleTime=on
  Memory1 : Memory  InitialCondition=model.T_1_Init  InheritSampleTime=on
  Saturation : Saturate  UpperLimit=1  LowerLimit=0
  Saturation1 : Saturate  UpperLimit=inf  LowerLimit=273
  To Workspace : ToWorkspace  VariableName=simT_1  SampleTime=-1
  To Workspace1 : ToWorkspace  VariableName=simx_r  SampleTime=-1
  T_e : Outport
  wires:
  [p_im] -> Divide/2
  [p_em] -> Divide/1
  Divide/1 -> [pai_e]
  Constant2/1 -> Divide1/2
  [q_in] -> Divide7/2, Divide2/1
  Constant6/1 -> Divide5/2, Divide3/1
  Constant5/1 -> Add5/2, Divide2/2
  Constant9/1 -> Add2/2
  Constant8/1 -> Add2/1
  Constant3/1 -> Add/1
  [W_f] -> Divide1/3, Add1/1
  [W_ei] -> Add1/2
  Add1/1 -> Divide1/4
  Divide1/1 -> [q_in]
  Add2/1 -> Math Function/2
  Constant7/1 -> Math Function/1
  Math Function/1 -> Divide19/2, Divide4/3
  Divide3/1 -> Divide4/2
  Divide2/1 -> Divide5/1, Divide4/1
  Divide4/1 -> Add3/2
  Constant4/1 -> Add5/1, Add3/1
  Add3/1 -> [x_p]
  Divide5/1 -> Add4/2
  Add4/1 -> Divide6/1
  Constant10/1 -> Divide6/2
  Add/1 -> Divide1/1
  Add5/1 -> Divide7/1
  Divide7/1 -> [t1]
  [t1] -> Divide8/1
  Divide6/1 -> Divide8/2
  Divide8/1 -> Add6/2
  Constant11/1 -> Add6/1
  Add6/1 -> [x_v]
  Constant14/1 -> Divide9/1
  Constant13/1 -> Divide9/2
  [pai_e] -> Math Function1/1
  Divide9/1 -> Gain/1, Math Function1/2
  [x_p] -> Math Function2/1
  Gain/1 -> Math Function2/2
  Math Function1/1 -> Divide10/1
  Math Function2/1 -> Divide10/2
  [x_v] -> Divide10/3
  Constant12/1 -> Divide10/4
  Constant15/1 -> Math Function4/1, Math Function6/1
  Math Function3/1 -> Divide16/2
  [pai_e] -> Math Function3/1
  Constant16/1 -> Add8/2, Divide11/2
  Constant17/1 -> Add8/1, Divide11/1, Add7/1
  Divide11/1 -> Add7/2
  Add7/1 -> Gain2/1, Math Function3/2
  [x_p] -> Math Function5/1
  Gain2/1 -> Math Function5/2
  Add8/1 -> Gain1/1, Math Function6/2
  Constant24/1 -> Add9/1
  Constant22/1 -> Divide13/1, Add9/2
  Add9/1 -> Divide12/1
  Constant20/1 -> Divide12/2
  Constant21/1 -> Divide13/2
  Divide12/1 -> Add10/1
  Divide13/1 -> Add10/2
  [q_in] -> Divide14/2
  Add10/1 -> Divide14/1
  Gain1/1 -> Math Function4/2
  Math Function4/1 -> Divide15/1
  Divide15/1 -> Add11/1
  Divide14/1 -> Add11/2
  Add11/1 -> Divide16/5
  Math Function6/1 -> Divide16/4
  Math Function5/1 -> Divide16/3
  Constant18/1 -> Divide16/1
  Divide16/1 -> [T_e], T_e/1
  Constant19/1 -> Add12/1
  Add12/1 -> Divide17/1
  Constant25/1 -> Divide17/2
  [T_e] -> Divide18/2
  Divide17/1 -> Add13/1
  Divide18/1 -> Add13/2
  Add13/1 -> Saturation1/1
  [T_1] -> Divide19/1, Divide3/2
  Divide19/1 -> Add4/1
  [T_1] -> Divide15/2
  [x_r] -> Add/2
  Divide10/1 -> Saturation/1
  Memory/1 -> To Workspace1/1, [x_r]
  Saturation/1 -> Memory/1
  Saturation1/1 -> Memory1/1
  Memory1/1 -> To Workspace/1, [T_1]
  [x_r] -> Divide18/1, Add12/2
